simulink model "NPC_grid_tied"  (R2020a)
settings: Solver=ode8  StartTime=0.0  StopTime=0.1  FixedStep=1e-6  RelTol=1e-3
libraries: powerlib x31, simulink x6
(part 1 of 2)
settings Model: Creator=Administrator  LastModifiedBy=captaincc
settings DataIOCC: ReturnWorkspaceOutputs=off
settings DebuggingCC: ArithmeticOperatorsInVariantConditions=warning
settings SFSimCC: CustomCodeUndefinedFunction=UseInterfaceOnly

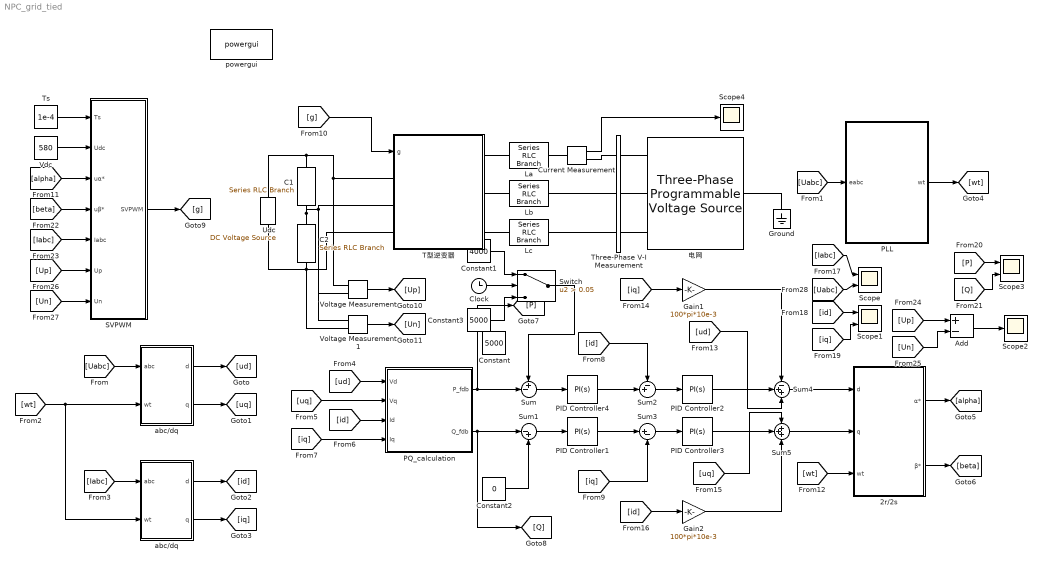
== system NPC_grid_tied ==
  2r/2s : Subsystem
  Add : Sum  Inputs=+-
  C1 : powerlib/Elements/Series RLC Branch  LConnTagsString=__new0  RConnTagsString=__new0  BranchType=RC  Resistance=1e-3  Inductance=1e-3  SetiL0=off  InitialCurrent=0  Capacitance=600e-6  Setx0=off  InitialVoltage=0  Measurements=None
  C2 : powerlib/Elements/Series RLC Branch  LConnTagsString=__new0  RConnTagsString=__new0  BranchType=RC  Resistance=1e-3  Inductance=1e-3  SetiL0=off  InitialCurrent=0  Capacitance=600e-6  Setx0=off  InitialVoltage=0  Measurements=None
  Clock : Clock
  Constant : Constant  Value=5000
  Constant1 : Constant  Value=4000
  Constant2 : Constant  Value=0
  Constant3 : Constant  Value=5000
  Current Measurement : powerlib/Measurements/Current Measurement  PhasorSimulation=off  OutputType=Complex  PSBequivalent=0
  Gain1 : Gain  Gain=100*pi*10e-3
  Gain2 : Gain  Gain=100*pi*10e-3
  Ground : powerlib/Elements/Ground  LConnTagsString=a
  La : powerlib/Elements/Series RLC Branch  LConnTagsString=__new0  RConnTagsString=__new0  BranchType=L  Resistance=1  Inductance=10e-3  SetiL0=off  InitialCurrent=0  Capacitance=1e-6  Setx0=off  InitialVoltage=0  Measurements=None
  Lb : powerlib/Elements/Series RLC Branch  LConnTagsString=__new0  RConnTagsString=__new0  BranchType=L  Resistance=1  Inductance=10e-3  SetiL0=off  InitialCurrent=0  Capacitance=1e-6  Setx0=off  InitialVoltage=0  Measurements=None
  Lc : powerlib/Elements/Series RLC Branch  LConnTagsString=__new0  RConnTagsString=__new0  BranchType=L  Resistance=1  Inductance=10e-3  SetiL0=off  InitialCurrent=0  Capacitance=1e-6  Setx0=off  InitialVoltage=0  Measurements=None
  PID Controller1 : simulink/Continuous/PID Controller  Controller=PI  Form=Parallel  TimeDomain=Continuous-time  UseExternalTs=off  SampleTime=-1  IntegratorMethod=Forward Euler  FilterMethod=Forward Euler  ControllerParametersSource=internal  P=0.0014  I=1.0395  D=0  UseFilter=on  N=100  TunerSelectOption=Transfer Function Based (PID Tuner App)  InitialConditionSource=internal  InitialConditionForIntegrator=0  InitialConditionForFilter=0  DifferentiatorICPrevScaledInput=0  ExternalReset=none  TrackingMode=off  Kt=1  LimitOutput=off  UpperSaturationLimit=inf  LowerSaturationLimit=-inf  LinearizeAsGain=on  AntiWindupMode=none  Kb=1  POutMin=[]  POutMax=[]  IOutMin=[]  IOutMax=[]  DOutMin=[]  DOutMax=[]  NOutMin=[]  NOutMax=[]  SumOutMin=[]  SumOutMax=[]  SaturationOutMin=[]  SaturationOutMax=[]  PParamMin=[]  PParamMax=[]  IParamMin=[]  IParamMax=[]  DParamMin=[]  DParamMax=[]  NParamMin=[]  NParamMax=[]  KbParamMin=[]  KbParamMax=[]  KtParamMin=[]  KtParamMax=[]  KbOutMin=[]  KbOutMax=[]  KtOutMin=[]  KtOutMax=[]  IntegratorOutMin=[]  IntegratorOutMax=[]  FilterOutMin=[]  FilterOutMax=[]  SumI1OutMin=[]  SumI1OutMax=[]  SumI2OutMin=[]  SumI2OutMax=[]  SumI3OutMin=[]  SumI3OutMax=[]  SumI4OutMin=[]  SumI4OutMax=[]  SumDOutMin=[]  SumDOutMax=[]  DifferentiatorOutMin=[]  DifferentiatorOutMax=[]  FilterDiffOutCoefMin=[]  FilterDiffOutCoefMax=[]  ReciprocalOutMin=[]  ReciprocalOutMax=[]  SumDenOutMin=[]  SumDenOutMax=[]  SumNumOutMin=[]  SumNumOutMax=[]  DivideOutMin=[]  DivideOutMax=[]  UdiffTsProdOutMin=[]  UdiffTsProdOutMax=[]  NTsProdOutMin=[]  NTsProdOutMax=[]  UintegralTsProdOutMin=[]  UintegralTsProdOutMax=[]  UngainTsProdOutMin=[]  UngainTsProdOutMax=[]  IntegratorContinuousStateAttributes=''  IntegratorStateMustResolveToSignalObject=off  IntegratorRTWStateStorageClass=Auto  FilterContinuousStateAttributes=''  FilterStateMustResolveToSignalObject=off  FilterRTWStateStorageClass=Auto  ParallelPVariant=InternalParameters  IdealPVariant=Disabled  IVariant=InternalParameters  DVariant=Disabled  IntegratorVariant=Continuous  SatVariant=Disabled  AWVariant=Passthrough  PCopyVariant=Disabled  TRVariant=Disabled  FdbkBlocksVariant=Forward  IdealPFdbkVariant=Disabled  SatFdbkVariant=Disabled  DerivativeFilterVariant=Disabled  NVariant=Disabled  NCopyVariant=Disabled_SignalSpec  FilterICVariant=Disabled  IntegratorICVariant=InternalICs  ExternalResetVariant=Disabled  TRSumVariant=Passthrough  SumFdbkVariant=Disabled  SumVariant=Sum_PI  TsampFilterVariant=InternalTs  TsampNgainVariant=Passthrough  TsampIntegralVariant=Passthrough
  PID Controller2 : simulink/Continuous/PID Controller  Controller=PI  Form=Parallel  TimeDomain=Continuous-time  UseExternalTs=off  SampleTime=-1  IntegratorMethod=Forward Euler  FilterMethod=Forward Euler  ControllerParametersSource=internal  P=33  I=333  D=0  UseFilter=on  N=100  TunerSelectOption=Transfer Function Based (PID Tuner App)  InitialConditionSource=internal  InitialConditionForIntegrator=0  InitialConditionForFilter=0  DifferentiatorICPrevScaledInput=0  ExternalReset=none  TrackingMode=off  Kt=1  LimitOutput=off  UpperSaturationLimit=inf  LowerSaturationLimit=-inf  LinearizeAsGain=on  AntiWindupMode=none  Kb=1  POutMin=[]  POutMax=[]  IOutMin=[]  IOutMax=[]  DOutMin=[]  DOutMax=[]  NOutMin=[]  NOutMax=[]  SumOutMin=[]  SumOutMax=[]  SaturationOutMin=[]  SaturationOutMax=[]  PParamMin=[]  PParamMax=[]  IParamMin=[]  IParamMax=[]  DParamMin=[]  DParamMax=[]  NParamMin=[]  NParamMax=[]  KbParamMin=[]  KbParamMax=[]  KtParamMin=[]  KtParamMax=[]  KbOutMin=[]  KbOutMax=[]  KtOutMin=[]  KtOutMax=[]  IntegratorOutMin=[]  IntegratorOutMax=[]  FilterOutMin=[]  FilterOutMax=[]  SumI1OutMin=[]  SumI1OutMax=[]  SumI2OutMin=[]  SumI2OutMax=[]  SumI3OutMin=[]  SumI3OutMax=[]  SumI4OutMin=[]  SumI4OutMax=[]  SumDOutMin=[]  SumDOutMax=[]  DifferentiatorOutMin=[]  DifferentiatorOutMax=[]  FilterDiffOutCoefMin=[]  FilterDiffOutCoefMax=[]  ReciprocalOutMin=[]  ReciprocalOutMax=[]  SumDenOutMin=[]  SumDenOutMax=[]  SumNumOutMin=[]  SumNumOutMax=[]  DivideOutMin=[]  DivideOutMax=[]  UdiffTsProdOutMin=[]  UdiffTsProdOutMax=[]  NTsProdOutMin=[]  NTsProdOutMax=[]  UintegralTsProdOutMin=[]  UintegralTsProdOutMax=[]  UngainTsProdOutMin=[]  UngainTsProdOutMax=[]  IntegratorContinuousStateAttributes=''  IntegratorStateMustResolveToSignalObject=off  IntegratorRTWStateStorageClass=Auto  FilterContinuousStateAttributes=''  FilterStateMustResolveToSignalObject=off  FilterRTWStateStorageClass=Auto  ParallelPVariant=InternalParameters  IdealPVariant=Disabled  IVariant=InternalParameters  DVariant=Disabled  IntegratorVariant=Continuous  SatVariant=Disabled  AWVariant=Passthrough  PCopyVariant=Disabled  TRVariant=Disabled  FdbkBlocksVariant=Forward  IdealPFdbkVariant=Disabled  SatFdbkVariant=Disabled  DerivativeFilterVariant=Disabled  NVariant=Disabled  NCopyVariant=Disabled_SignalSpec  FilterICVariant=Disabled  IntegratorICVariant=InternalICs  ExternalResetVariant=Disabled  TRSumVariant=Passthrough  SumFdbkVariant=Disabled  SumVariant=Sum_PI  TsampFilterVariant=InternalTs  TsampNgainVariant=Passthrough  TsampIntegralVariant=Passthrough
  PID Controller3 : simulink/Continuous/PID Controller  Controller=PI  Form=Parallel  TimeDomain=Continuous-time  UseExternalTs=off  SampleTime=-1  IntegratorMethod=Forward Euler  FilterMethod=Forward Euler  ControllerParametersSource=internal  P=33  I=333  D=0  UseFilter=on  N=100  TunerSelectOption=Transfer Function Based (PID Tuner App)  InitialConditionSource=internal  InitialConditionForIntegrator=0  InitialConditionForFilter=0  DifferentiatorICPrevScaledInput=0  ExternalReset=none  TrackingMode=off  Kt=1  LimitOutput=off  UpperSaturationLimit=inf  LowerSaturationLimit=-inf  LinearizeAsGain=on  AntiWindupMode=none  Kb=1  POutMin=[]  POutMax=[]  IOutMin=[]  IOutMax=[]  DOutMin=[]  DOutMax=[]  NOutMin=[]  NOutMax=[]  SumOutMin=[]  SumOutMax=[]  SaturationOutMin=[]  SaturationOutMax=[]  PParamMin=[]  PParamMax=[]  IParamMin=[]  IParamMax=[]  DParamMin=[]  DParamMax=[]  NParamMin=[]  NParamMax=[]  KbParamMin=[]  KbParamMax=[]  KtParamMin=[]  KtParamMax=[]  KbOutMin=[]  KbOutMax=[]  KtOutMin=[]  KtOutMax=[]  IntegratorOutMin=[]  IntegratorOutMax=[]  FilterOutMin=[]  FilterOutMax=[]  SumI1OutMin=[]  SumI1OutMax=[]  SumI2OutMin=[]  SumI2OutMax=[]  SumI3OutMin=[]  SumI3OutMax=[]  SumI4OutMin=[]  SumI4OutMax=[]  SumDOutMin=[]  SumDOutMax=[]  DifferentiatorOutMin=[]  DifferentiatorOutMax=[]  FilterDiffOutCoefMin=[]  FilterDiffOutCoefMax=[]  ReciprocalOutMin=[]  ReciprocalOutMax=[]  SumDenOutMin=[]  SumDenOutMax=[]  SumNumOutMin=[]  SumNumOutMax=[]  DivideOutMin=[]  DivideOutMax=[]  UdiffTsProdOutMin=[]  UdiffTsProdOutMax=[]  NTsProdOutMin=[]  NTsProdOutMax=[]  UintegralTsProdOutMin=[]  UintegralTsProdOutMax=[]  UngainTsProdOutMin=[]  UngainTsProdOutMax=[]  IntegratorContinuousStateAttributes=''  IntegratorStateMustResolveToSignalObject=off  IntegratorRTWStateStorageClass=Auto  FilterContinuousStateAttributes=''  FilterStateMustResolveToSignalObject=off  FilterRTWStateStorageClass=Auto  ParallelPVariant=InternalParameters  IdealPVariant=Disabled  IVariant=InternalParameters  DVariant=Disabled  IntegratorVariant=Continuous  SatVariant=Disabled  AWVariant=Passthrough  PCopyVariant=Disabled  TRVariant=Disabled  FdbkBlocksVariant=Forward  IdealPFdbkVariant=Disabled  SatFdbkVariant=Disabled  DerivativeFilterVariant=Disabled  NVariant=Disabled  NCopyVariant=Disabled_SignalSpec  FilterICVariant=Disabled  IntegratorICVariant=InternalICs  ExternalResetVariant=Disabled  TRSumVariant=Passthrough  SumFdbkVariant=Disabled  SumVariant=Sum_PI  TsampFilterVariant=InternalTs  TsampNgainVariant=Passthrough  TsampIntegralVariant=Passthrough
  PID Controller4 : simulink/Continuous/PID Controller  Controller=PI  Form=Parallel  TimeDomain=Continuous-time  UseExternalTs=off  SampleTime=-1  IntegratorMethod=Forward Euler  FilterMethod=Forward Euler  ControllerParametersSource=internal  P=0.0014  I=1.0395  D=0  UseFilter=on  N=100  TunerSelectOption=Transfer Function Based (PID Tuner App)  InitialConditionSource=internal  InitialConditionForIntegrator=0  InitialConditionForFilter=0  DifferentiatorICPrevScaledInput=0  ExternalReset=none  TrackingMode=off  Kt=1  LimitOutput=off  UpperSaturationLimit=inf  LowerSaturationLimit=-inf  LinearizeAsGain=on  AntiWindupMode=none  Kb=1  POutMin=[]  POutMax=[]  IOutMin=[]  IOutMax=[]  DOutMin=[]  DOutMax=[]  NOutMin=[]  NOutMax=[]  SumOutMin=[]  SumOutMax=[]  SaturationOutMin=[]  SaturationOutMax=[]  PParamMin=[]  PParamMax=[]  IParamMin=[]  IParamMax=[]  DParamMin=[]  DParamMax=[]  NParamMin=[]  NParamMax=[]  KbParamMin=[]  KbParamMax=[]  KtParamMin=[]  KtParamMax=[]  KbOutMin=[]  KbOutMax=[]  KtOutMin=[]  KtOutMax=[]  IntegratorOutMin=[]  IntegratorOutMax=[]  FilterOutMin=[]  FilterOutMax=[]  SumI1OutMin=[]  SumI1OutMax=[]  SumI2OutMin=[]  SumI2OutMax=[]  SumI3OutMin=[]  SumI3OutMax=[]  SumI4OutMin=[]  SumI4OutMax=[]  SumDOutMin=[]  SumDOutMax=[]  DifferentiatorOutMin=[]  DifferentiatorOutMax=[]  FilterDiffOutCoefMin=[]  FilterDiffOutCoefMax=[]  ReciprocalOutMin=[]  ReciprocalOutMax=[]  SumDenOutMin=[]  SumDenOutMax=[]  SumNumOutMin=[]  SumNumOutMax=[]  DivideOutMin=[]  DivideOutMax=[]  UdiffTsProdOutMin=[]  UdiffTsProdOutMax=[]  NTsProdOutMin=[]  NTsProdOutMax=[]  UintegralTsProdOutMin=[]  UintegralTsProdOutMax=[]  UngainTsProdOutMin=[]  UngainTsProdOutMax=[]  IntegratorContinuousStateAttributes=''  IntegratorStateMustResolveToSignalObject=off  IntegratorRTWStateStorageClass=Auto  FilterContinuousStateAttributes=''  FilterStateMustResolveToSignalObject=off  FilterRTWStateStorageClass=Auto  ParallelPVariant=InternalParameters  IdealPVariant=Disabled  IVariant=InternalParameters  DVariant=Disabled  IntegratorVariant=Continuous  SatVariant=Disabled  AWVariant=Passthrough  PCopyVariant=Disabled  TRVariant=Disabled  FdbkBlocksVariant=Forward  IdealPFdbkVariant=Disabled  SatFdbkVariant=Disabled  DerivativeFilterVariant=Disabled  NVariant=Disabled  NCopyVariant=Disabled_SignalSpec  FilterICVariant=Disabled  IntegratorICVariant=InternalICs  ExternalResetVariant=Disabled  TRSumVariant=Passthrough  SumFdbkVariant=Disabled  SumVariant=Sum_PI  TsampFilterVariant=InternalTs  TsampNgainVariant=Passthrough  TsampIntegralVariant=Passthrough
  PLL : Subsystem
  PQ_calculation : Subsystem
  SVPWM : Subsystem
  Scope : Scope  NumInputPorts=2
  Scope1 : Scope  NumInputPorts=2
  Scope2 : Scope
  Scope3 : Scope  NumInputPorts=2
  Scope4 : Scope
  Sum : Sum  Inputs=+-|
  Sum1 : Sum  Inputs=|-+
  Sum2 : Sum  Inputs=-+|
  Sum3 : Sum  Inputs=|+-
  Sum4 : Sum  Inputs=-++
  Sum5 : Sum  Inputs=+++
  Switch : Switch  Criteria=u2 > Threshold  Threshold=0.05
  Three-Phase V-I Measurement : powerlib/Measurements/Three-Phase V-I Measurement  VoltageMeasurement=phase-to-ground  SetLabelV=on  LabelV=Uabc  Vpu=off  VpuLL=off  CurrentMeasurement=yes  SetLabelI=on  LabelI=Iabc  Ipu=off  Pbase=100e6  Vbase=500e3  OutputType=Complex  PhasorSimulation=off  PSBequivalent=0
  Ts : Constant  Value=1e-4
  T型逆变器 : Subsystem
  Udc : powerlib/Electrical Sources/DC Voltage Source  Amplitude=580  Measurements=None
  Vdc : Constant  Value=580
  Voltage Measurement : powerlib/Measurements/Voltage Measurement  PhasorSimulation=off  OutputType=Complex  PSBequivalent=0
  Voltage Measurement1 : powerlib/Measurements/Voltage Measurement  PhasorSimulation=off  OutputType=Complex  PSBequivalent=0
  abc/dq : Subsystem
  "abc/dq " : Subsystem
  powergui : powerlib/powergui  Priority=1  SimulationMode=Continuous  SampleTime=1e-6  frequency=60  Iterations=50  frequencyindice=0  Pbase=100e6  ErrMax=1e-4  UnitsV=kV  UnitsW=MW  buscounter=0  FunctionMessages=off  echomessages=off  EnableUseOfTLC=off  CurrentSourceSwitches=off  DisableSnubberDevices=off  DisableRonSwitches=off  DisableVfSwitches=off  DisplayEquations=off  AutomaticDiscreteSolvers=off  SolverType=Tustin/Backward Euler (TBE)  Interpol=off  ExternalGateDelay=off  methode=off  Ts=100  x0status=blocks  SPID=off  SwTol=0  HookPort=off  NonlinearTolerance=1e-4  nMaxIteration=100  ContinueOnMaxIteration=off  RestoreLinks=warning  ResistiveCurrentMeasurement=off  Frange=[0:2:500]  Ylog=off  Xlog=on  ShowGrid=off  save=off  variable=ZData  structure=Ia  ZoomFFT=off  StartTime=0.03  cycles=2  DisplayStyle=1  fundamental=50  FreqAxis=off  MaxFrequency=1000  frequencyindicesteady=1  RmsSteady=1  display=off
  电网 : powerlib/Electrical Sources/Three-Phase Programmable Voltage Source  PositiveSequence=[220*sqrt(3) 0 50]  VariationEntity=None  VariationType=Step  VariationTypeAlt=Step  VariationStep=0.5  VariationRate=10  VariationMagnitude=0.3  VariationFrequency=2  VariationTiming=[1 2]  VariationPhaseA=off  Amplitudes=[1 0.8 1.2 1.0]  TimeValues=[0 0.1 0.15 0.2]  HarmonicGeneration=off  HarmonicA=[3 0.2 -25 0]  HarmonicB=[2 0.15 35 2]  Timing="[0.05  3]"  BusType=swing  Pref=10000  Qref=0  Qmin=-inf  Qmax=inf
  wires:
  [Uabc] -> PLL/1(eabc)
  PLL/1(wt) -> [wt]
  [ud] -> PQ_calculation/1(Vd)
  [uq] -> PQ_calculation/2(Vq)
  [id] -> PQ_calculation/3(Id)
  [iq] -> PQ_calculation/4(Iq)
  PQ_calculation/2(Q_fdb) -> Sum1/1, [Q]
  PQ_calculation/1(P_fdb) -> Sum/2, [P]
  Constant2/1 -> Sum1/2
  PID Controller4/1 -> Sum2/2
  PID Controller1/1 -> Sum3/1
  [id] -> Sum2/1
  [iq] -> Sum3/2
  Sum2/1 -> PID Controller2/1
  Sum3/1 -> PID Controller3/1
  [wt] -> 2r/2s/3(wt)
  2r/2s/1(α*) -> [alpha]
  2r/2s/2(β*) -> [beta]
  [wt] -> "abc/dq "/2(wt), abc/dq/2(wt)
  [Iabc] -> "abc/dq "/1(abc)
  abc/dq/2(q) -> [uq]
  abc/dq/1(d) -> [ud]
  [Uabc] -> abc/dq/1(abc)
  "abc/dq "/2(q) -> [iq]
  "abc/dq "/1(d) -> [id]
  [ud] -> Sum4/3
  PID Controller2/1 -> Sum4/2
  [iq] -> Gain1/1
  Gain1/1 -> Sum4/1
  PID Controller3/1 -> Sum5/2
  Gain2/1 -> Sum5/3
  [uq] -> Sum5/1
  [id] -> Gain2/1
  Current Measurement/1 -> Scope4/1
  [id] -> Scope1/1
  [iq] -> Scope1/2
  [P] -> Scope3/1
  [Q] -> Scope3/2
  Sum4/1 -> 2r/2s/1(d)
  Sum5/1 -> 2r/2s/2(q)
  Sum/1 -> PID Controller4/1
  Sum1/1 -> PID Controller1/1
  Ts/1 -> SVPWM/1(Ts)
  Vdc/1 -> SVPWM/2(Udc)
  [g] -> T型逆变器/1(g)
  SVPWM/1(SVPWM) -> [g]
  [alpha] -> SVPWM/3(uα*)
  [beta] -> SVPWM/4(uβ*)
  [Iabc] -> Scope/1
  [Iabc] -> SVPWM/5(Iabc)
  Voltage Measurement/1 -> [Up]
  Voltage Measurement1/1 -> [Un]
  [Up] -> Add/1
  [Un] -> Add/2
  Add/1 -> Scope2/1
  [Up] -> SVPWM/6(Up)
  [Un] -> SVPWM/7(Un)
  [Uabc] -> Scope/2
  Switch/1 -> Sum/1
  Clock/1 -> Switch/2
  Constant3/1 -> Switch/3
  Constant1/1 -> Switch/1
  connections:
  T型逆变器/RConn1 -- La/LConn1
  电网/RConn1 -- Three-Phase V-I Measurement/RConn1
  Three-Phase V-I Measurement/LConn2 -- Lb/RConn1
  Three-Phase V-I Measurement/LConn3 -- Lc/RConn1
  T型逆变器/RConn2 -- Lb/LConn1
  T型逆变器/RConn3 -- Lc/LConn1
  电网/RConn2 -- Three-Phase V-I Measurement/RConn2
  电网/RConn3 -- Three-Phase V-I Measurement/RConn3
  Ground/LConn1 -- 电网/LConn1
  Current Measurement/LConn1 -- La/RConn1
  Current Measurement/RConn1 -- Three-Phase V-I Measurement/LConn1
  Udc/LConn1 -- Voltage Measurement1/LConn2 -- C2/RConn1 -- T型逆变器/LConn3
  C2/LConn1 -- Voltage Measurement1/LConn1 -- Voltage Measurement/LConn2 -- T型逆变器/LConn2 -- C1/RConn1
  C1/LConn1 -- Udc/RConn1 -- Voltage Measurement/LConn1 -- T型逆变器/LConn1

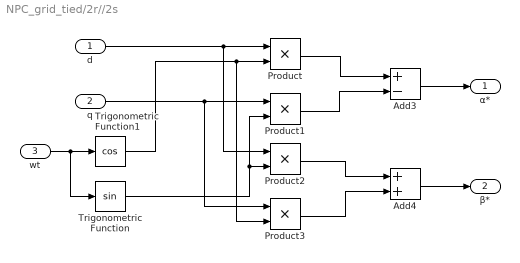
== system NPC_grid_tied/2r//2s ==
  d : Inport
  q : Inport  Port=2
  wt : Inport  Port=3
  Add3 : Sum  Inputs=+-
  Add4 : Sum
  Product{,1..3} (4 alike) : Product
  Trigonometric Function : Trigonometry
  Trigonometric Function1 : Trigonometry  Operator=cos
  α* : Outport  VectorParamsAs1DForOutWhenUnconnected=off
  β* : Outport  Port=2  VectorParamsAs1DForOutWhenUnconnected=off
  wires:
  q/1 -> Product3/1, Product1/1
  Trigonometric Function/1 -> Product1/2, Product2/2
  Trigonometric Function1/1 -> Product3/2, Product/2
  d/1 -> Product2/1, Product/1
  Product2/1 -> Add4/1
  Product/1 -> Add3/1
  Product1/1 -> Add3/2
  Product3/1 -> Add4/2
  Add3/1 -> α*/1
  Add4/1 -> β*/1
  wt/1 -> Trigonometric Function/1, Trigonometric Function1/1

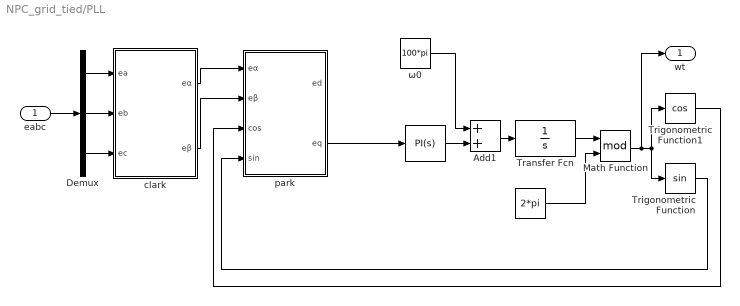
== system NPC_grid_tied/PLL ==
  eabc : Inport
  " " : Constant  Value=2*pi
  " " : simulink/Continuous/PID Controller  Controller=PI  Form=Parallel  TimeDomain=Continuous-time  UseExternalTs=off  SampleTime=-1  IntegratorMethod=Trapezoidal  FilterMethod=Forward Euler  ControllerParametersSource=internal  P=0.826  I=82.7  D=0  UseFilter=on  N=100  TunerSelectOption=Transfer Function Based (PID Tuner App)  InitialConditionSource=internal  InitialConditionForIntegrator=0  InitialConditionForFilter=0  DifferentiatorICPrevScaledInput=0  ExternalReset=none  TrackingMode=off  Kt=1  LimitOutput=off  UpperSaturationLimit=inf  LowerSaturationLimit=-inf  LinearizeAsGain=off  AntiWindupMode=none  Kb=1  POutMin=[]  POutMax=[]  IOutMin=[]  IOutMax=[]  DOutMin=[]  DOutMax=[]  NOutMin=[]  NOutMax=[]  SumOutMin=[]  SumOutMax=[]  SaturationOutMin=[]  SaturationOutMax=[]  PParamMin=[]  PParamMax=[]  IParamMin=[]  IParamMax=[]  DParamMin=[]  DParamMax=[]  NParamMin=[]  NParamMax=[]  KbParamMin=[]  KbParamMax=[]  KtParamMin=[]  KtParamMax=[]  KbOutMin=[]  KbOutMax=[]  KtOutMin=[]  KtOutMax=[]  IntegratorOutMin=[]  IntegratorOutMax=[]  FilterOutMin=[]  FilterOutMax=[]  SumI1OutMin=[]  SumI1OutMax=[]  SumI2OutMin=[]  SumI2OutMax=[]  SumI3OutMin=[]  SumI3OutMax=[]  SumI4OutMin=[]  SumI4OutMax=[]  SumDOutMin=[]  SumDOutMax=[]  DifferentiatorOutMin=[]  DifferentiatorOutMax=[]  FilterDiffOutCoefMin=[]  FilterDiffOutCoefMax=[]  ReciprocalOutMin=[]  ReciprocalOutMax=[]  SumDenOutMin=[]  SumDenOutMax=[]  SumNumOutMin=[]  SumNumOutMax=[]  DivideOutMin=[]  DivideOutMax=[]  UdiffTsProdOutMin=[]  UdiffTsProdOutMax=[]  NTsProdOutMin=[]  NTsProdOutMax=[]  UintegralTsProdOutMin=[]  UintegralTsProdOutMax=[]  UngainTsProdOutMin=[]  UngainTsProdOutMax=[]  IntegratorContinuousStateAttributes=''  IntegratorStateMustResolveToSignalObject=off  IntegratorRTWStateStorageClass=Auto  FilterContinuousStateAttributes=''  FilterStateMustResolveToSignalObject=off  FilterRTWStateStorageClass=Auto  ParallelPVariant=InternalParameters  IdealPVariant=Disabled  IVariant=InternalParameters  DVariant=Disabled  IntegratorVariant=Continuous  SatVariant=Disabled  AWVariant=Passthrough  PCopyVariant=Disabled  TRVariant=Disabled  FdbkBlocksVariant=Forward  IdealPFdbkVariant=Disabled  SatFdbkVariant=Disabled  DerivativeFilterVariant=Disabled  NVariant=Disabled  NCopyVariant=Disabled_SignalSpec  FilterICVariant=Disabled  IntegratorICVariant=InternalICs  ExternalResetVariant=Disabled  TRSumVariant=Passthrough  SumFdbkVariant=Disabled  SumVariant=Sum_PI  TsampFilterVariant=InternalTs  TsampNgainVariant=Passthrough  TsampIntegralVariant=Passthrough
  Add1 : Sum
  Demux : Demux  Outputs=3
  Math Function : Math  Operator=mod  SignedPower=on  SaturateOnIntegerOverflow=on
  Transfer Fcn : TransferFcn  Denominator=[1 0]
  Trigonometric Function : Trigonometry
  Trigonometric Function1 : Trigonometry  Operator=cos
  clark : Subsystem
  park : Subsystem
  ω0 : Constant  Value=100*pi
  wt : Outport  VectorParamsAs1DForOutWhenUnconnected=off
  wires:
  Demux/2 -> clark/2(eb)
  Demux/1 -> clark/1(ea)
  Trigonometric Function/1 -> park/4(sin)
  clark/1(eα) -> park/1(eα)
  Trigonometric Function1/1 -> park/3(cos)
  Transfer Fcn/1 -> Math Function/1
  " "/1 -> Add1/2
  ω0/1 -> Add1/1
  Add1/1 -> Transfer Fcn/1
  clark/2(eβ) -> park/2(eβ)
  Demux/3 -> clark/3(ec)
  eabc/1 -> Demux/1
  park/2(eq) -> " "/1
  " "/1 -> Math Function/2
  Math Function/1 -> wt/1, Trigonometric Function/1, Trigonometric Function1/1

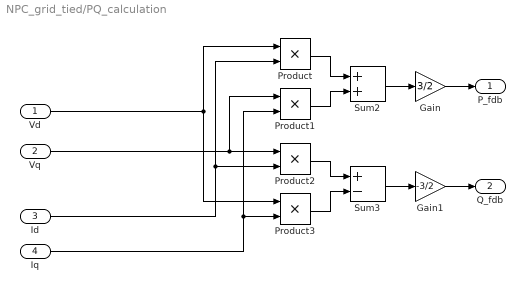
== system NPC_grid_tied/PQ_calculation ==
  Vd : Inport
  Vq : Inport  Port=2
  Id : Inport  Port=3
  Iq : Inport  Port=4
  Gain : Gain  Gain=3/2
  Gain1 : Gain  Gain=-3/2
  Product{,1..3} (4 alike) : Product
  Sum2 : Sum
  Sum3 : Sum  Inputs=+-
  P_fdb : Outport  VectorParamsAs1DForOutWhenUnconnected=off
  Q_fdb : Outport  Port=2  VectorParamsAs1DForOutWhenUnconnected=off
  wires:
  Product2/1 -> Sum3/1
  Iq/1 -> Product3/2, Product1/2
  Product3/1 -> Sum3/2
  Vq/1 -> Product1/1, Product2/1
  Id/1 -> Product2/2, Product/2
  Product/1 -> Sum2/1
  Vd/1 -> Product3/1, Product/1
  Product1/1 -> Sum2/2
  Gain/1 -> P_fdb/1
  Sum2/1 -> Gain/1
  Gain1/1 -> Q_fdb/1
  Sum3/1 -> Gain1/1

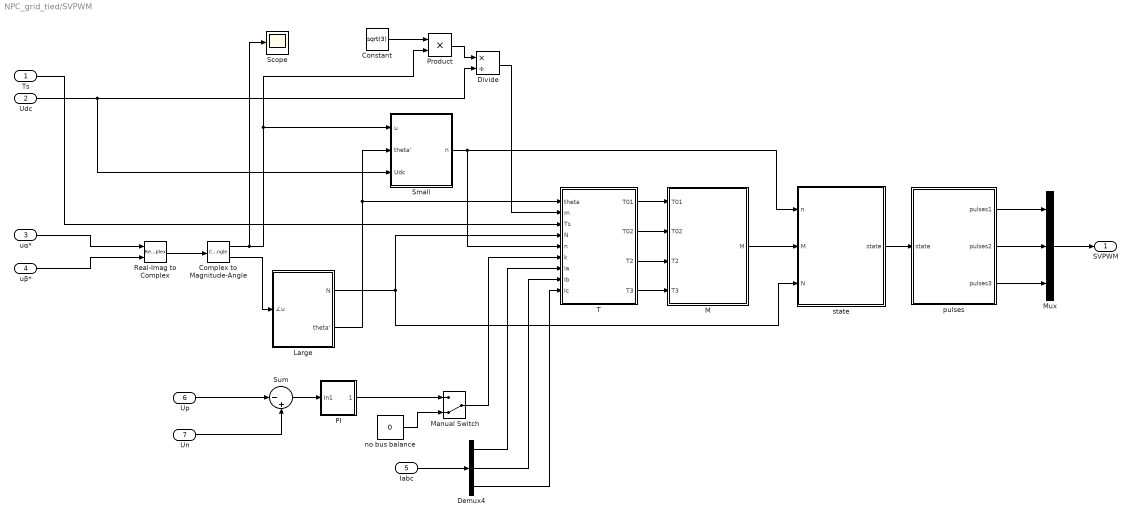
== system NPC_grid_tied/SVPWM ==
  Ts : Inport
  Udc : Inport  Port=2
  uα* : Inport  Port=3
  uβ* : Inport  Port=4
  Iabc : Inport  Port=5
  Up : Inport  Port=6
  Un : Inport  Port=7
  Complex to Magnitude-Angle : ComplexToMagnitudeAngle
  Constant : Constant  Value=sqrt(3)
  Demux4 : Demux  Outputs=3
  Divide : Product  Inputs=*/
  Large : Subsystem
  M : Subsystem
  Manual Switch : ManualSwitch  CurrentSetting=0
  Mux : Mux  Inputs=3
  PI : Subsystem
  Product : Product
  Real-Imag to Complex : RealImagToComplex
  Scope : Scope
  Small : Subsystem
  Sum : Sum  Inputs=|-+
  T : MATLAB Function  TreatAsAtomicUnit=on
  no bus balance : Constant  Value=0
  pulses : Subsystem
  state : Subsystem
  SVPWM : Outport  VectorParamsAs1DForOutWhenUnconnected=off
  wires:
  Udc/1 -> Divide/2, Small/3(Udc)
  Large/2(theta') -> T/1(theta), Small/2(theta')
  Product/1 -> Divide/1
  Complex to Magnitude-Angle/2 -> Large/1(∠u)
  Complex to Magnitude-Angle/1 -> Scope/1, Product/2, Small/1(u)
  Constant/1 -> Product/1
  pulses/1(pulses1) -> Mux/1
  pulses/2(pulses2) -> Mux/2
  pulses/3(pulses3) -> Mux/3
  state/1(state) -> pulses/1(state)
  Mux/1 -> SVPWM/1
  Real-Imag to Complex/1 -> Complex to Magnitude-Angle/1
  uα*/1 -> Real-Imag to Complex/1
  uβ*/1 -> Real-Imag to Complex/2
  Ts/1 -> T/3(Ts)
  PI/1(Out1) -> Manual Switch/1
  Demux4/1 -> T/7(Ia)
  Manual Switch/1 -> T/6(k)
  Large/1(N) -> T/4(N), state/3(N)
  T/1(T01) -> M/1(T01)
  Small/1(n) -> T/5(n), state/1(n)
  Divide/1 -> T/2(m)
  Demux4/3 -> T/9(Ic)
  Iabc/1 -> Demux4/1
  T/2(T02) -> M/2(T02)
  T/3(T2) -> M/3(T2)
  no bus balance/1 -> Manual Switch/2
  Demux4/2 -> T/8(Ib)
  T/4(T3) -> M/4(T3)
  M/1(M) -> state/2(M)
  Sum/1 -> PI/1(In1)
  Up/1 -> Sum/1
  Un/1 -> Sum/2

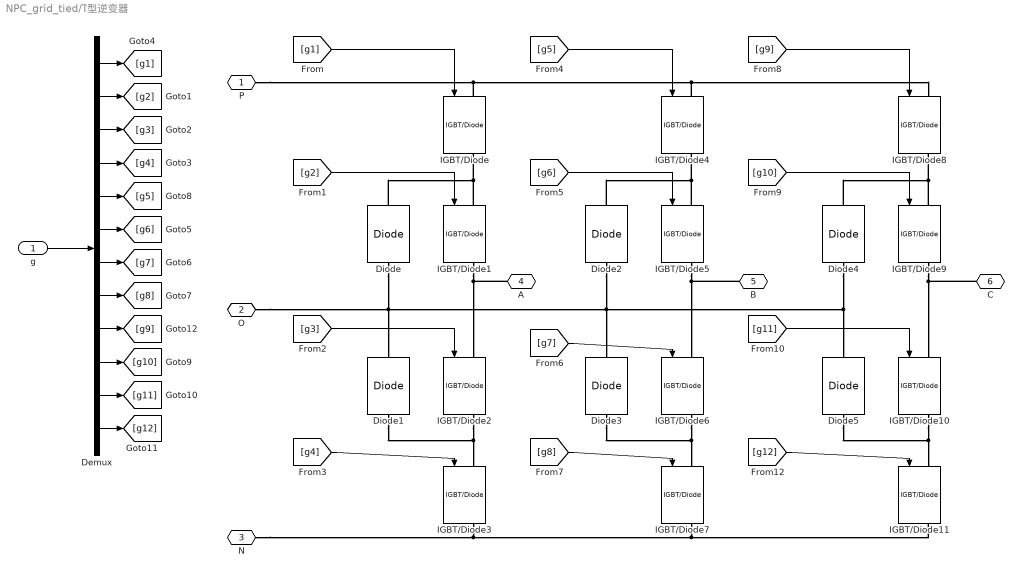
== system NPC_grid_tied/T型逆变器 ==
  g : Inport
  Demux : Demux  Outputs=12
  Diode{,1..5} (6 alike) : powerlib/Power Electronics/Diode  Ron=0.001  Lon=0  Vf=0.8  IC=0  UseSnubber=0  Rs=500  Cs=250e-9  Measurements=off
  IGBT/Diode{,1..11} (12 alike) : powerlib/Power Electronics/IGBT//Diode  Ron=1e-3  Rs=1e5  Cs=inf  Measurements=on
  P : PMIOPort  Side=Left
  O : PMIOPort  Port=2  Side=Left
  N : PMIOPort  Port=3  Side=Left
  A : PMIOPort  Port=4  Side=Right
  B : PMIOPort  Port=5  Side=Right
  C : PMIOPort  Port=6  Side=Right
  wires:
  Demux/1 -> [g1]
  Demux/2 -> [g2]
  Demux/3 -> [g3]
  Demux/4 -> [g4]
  Demux/5 -> [g5]
  Demux/6 -> [g6]
  Demux/7 -> [g7]
  Demux/8 -> [g8]
  Demux/9 -> [g9]
  Demux/10 -> [g10]
  Demux/11 -> [g11]
  Demux/12 -> [g12]
  [g1] -> IGBT/Diode/1
  [g2] -> IGBT/Diode1/1
  [g3] -> IGBT/Diode2/1
  [g4] -> IGBT/Diode3/1
  [g5] -> IGBT/Diode4/1
  [g6] -> IGBT/Diode5/1
  [g7] -> IGBT/Diode6/1
  [g8] -> IGBT/Diode7/1
  [g9] -> IGBT/Diode8/1
  [g10] -> IGBT/Diode9/1
  [g11] -> IGBT/Diode10/1
  [g12] -> IGBT/Diode11/1
  g/1 -> Demux/1
  connections:
  IGBT/Diode1/LConn1 -- Diode/RConn1 -- IGBT/Diode/RConn1
  IGBT/Diode1/RConn1 -- A/RConn1 -- IGBT/Diode2/LConn1
  IGBT/Diode2/RConn1 -- Diode1/LConn1 -- IGBT/Diode3/LConn1
  IGBT/Diode6/RConn1 -- Diode3/LConn1 -- IGBT/Diode7/LConn1
  IGBT/Diode5/LConn1 -- Diode2/RConn1 -- IGBT/Diode4/RConn1
  IGBT/Diode5/RConn1 -- IGBT/Diode6/LConn1 -- B/RConn1
  IGBT/Diode10/RConn1 -- Diode5/LConn1 -- IGBT/Diode11/LConn1
  IGBT/Diode9/LConn1 -- Diode4/RConn1 -- IGBT/Diode8/RConn1
  IGBT/Diode9/RConn1 -- C/RConn1 -- IGBT/Diode10/LConn1
  Diode/LConn1 -- Diode5/RConn1 -- Diode4/LConn1 -- Diode2/LConn1 -- Diode3/RConn1 -- O/RConn1 -- Diode1/RConn1
  IGBT/Diode/LConn1 -- P/RConn1 -- IGBT/Diode4/LConn1 -- IGBT/Diode8/LConn1
  IGBT/Diode3/RConn1 -- IGBT/Diode7/RConn1 -- IGBT/Diode11/RConn1 -- N/RConn1

== system NPC_grid_tied/abc//dq ==
  abc : Inport
  wt : Inport  Port=2
  Demux : Demux  Outputs=3
  Trigonometric Function : Trigonometry
  Trigonometric Function1 : Trigonometry  Operator=cos
  clark : Subsystem
  park : Subsystem
  d : Outport  VectorParamsAs1DForOutWhenUnconnected=off
  q : Outport  Port=2  VectorParamsAs1DForOutWhenUnconnected=off
  wires:
  Demux/1 -> clark/1(ea)
  clark/1(eα) -> park/1(eα)
  Demux/2 -> clark/2(eb)
  Trigonometric Function1/1 -> park/3(cos)
  wt/1 -> Trigonometric Function/1, Trigonometric Function1/1
  Demux/3 -> clark/3(ec)
  clark/2(eβ) -> park/2(eβ)
  park/2(eq) -> q/1
  park/1(ed) -> d/1
  abc/1 -> Demux/1
  Trigonometric Function/1 -> park/4(sin)

== system NPC_grid_tied/abc//dq  ==
  abc : Inport
  wt : Inport  Port=2
  Demux : Demux  Outputs=3
  Trigonometric Function : Trigonometry
  Trigonometric Function1 : Trigonometry  Operator=cos
  clark : Subsystem
  park : Subsystem
  d : Outport  VectorParamsAs1DForOutWhenUnconnected=off
  q : Outport  Port=2  VectorParamsAs1DForOutWhenUnconnected=off
  wires:
  Demux/1 -> clark/1(ea)
  clark/1(eα) -> park/1(eα)
  Demux/2 -> clark/2(eb)
  Trigonometric Function1/1 -> park/3(cos)
  wt/1 -> Trigonometric Function/1, Trigonometric Function1/1
  Demux/3 -> clark/3(ec)
  clark/2(eβ) -> park/2(eβ)
  park/2(eq) -> q/1
  park/1(ed) -> d/1
  abc/1 -> Demux/1
  Trigonometric Function/1 -> park/4(sin)

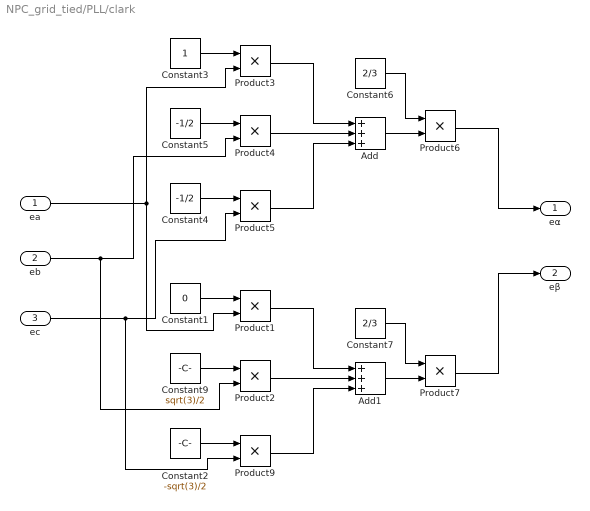
== system NPC_grid_tied/PLL/clark ==
  ea : Inport
  eb : Inport  Port=2
  ec : Inport  Port=3
  Add : Sum  Inputs=+++
  Add1 : Sum  Inputs=+++
  Constant1 : Constant  Value=0
  Constant2 : Constant  Value=-sqrt(3)/2
  Constant3 : Constant
  Constant4 : Constant  Value=-1/2
  Constant5 : Constant  Value=-1/2
  Constant6 : Constant  Value=2/3
  Constant7 : Constant  Value=2/3
  Constant9 : Constant  Value=sqrt(3)/2
  Product{1..7,9} (8 alike) : Product
  eα : Outport  VectorParamsAs1DForOutWhenUnconnected=off
  eβ : Outport  Port=2  VectorParamsAs1DForOutWhenUnconnected=off
  wires:
  Product5/1 -> Add/3
  eb/1 -> Product2/2, Product4/2
  Add1/1 -> Product7/2
  Constant7/1 -> Product7/1
  Product2/1 -> Add1/2
  Product4/1 -> Add/2
  Add/1 -> Product6/2
  Product6/1 -> eα/1
  Constant3/1 -> Product3/1
  Constant5/1 -> Product4/1
  ec/1 -> Product9/2, Product5/2
  ea/1 -> Product3/2, Product1/2
  Constant4/1 -> Product5/1
  Constant6/1 -> Product6/1
  Constant9/1 -> Product2/1
  Product3/1 -> Add/1
  Constant2/1 -> Product9/1
  Product9/1 -> Add1/3
  Product1/1 -> Add1/1
  Product7/1 -> eβ/1
  Constant1/1 -> Product1/1

== system NPC_grid_tied/PLL/park ==
  eα : Inport
  eβ : Inport  Port=2
  cos : Inport  Port=3
  sin : Inport  Port=4
  Add : Sum
  Add2 : Sum  Inputs=-+
  Product{,1..3} (4 alike) : Product
  ed : Outport  VectorParamsAs1DForOutWhenUnconnected=off
  eq : Outport  Port=2  VectorParamsAs1DForOutWhenUnconnected=off
  wires:
  Add2/1 -> eq/1
  Add/1 -> ed/1
  eα/1 -> Product2/1, Product/1
  cos/1 -> Product3/2, Product/2
  eβ/1 -> Product3/1, Product1/1
  sin/1 -> Product2/2, Product1/2
  Product/1 -> Add/1
  Product1/1 -> Add/2
  Product2/1 -> Add2/1
  Product3/1 -> Add2/2

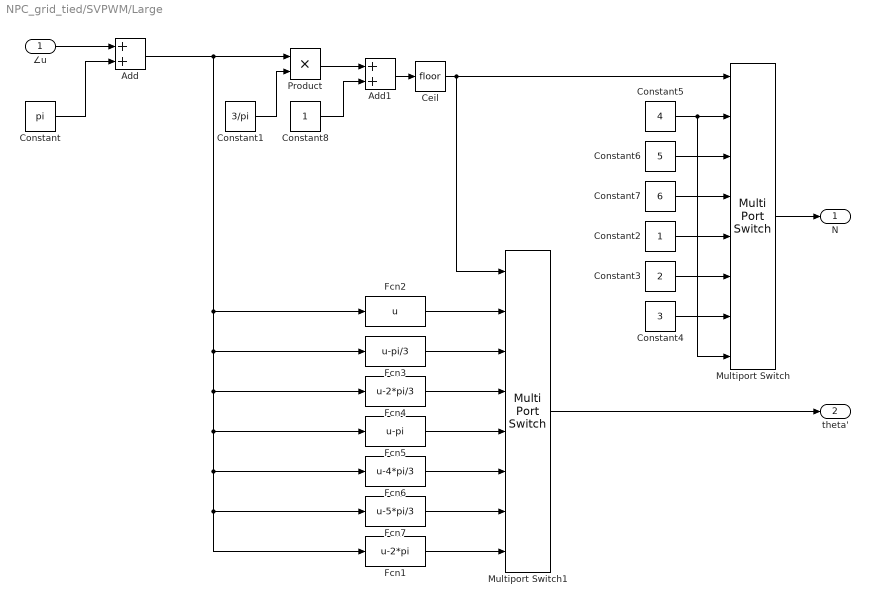
== system NPC_grid_tied/SVPWM/Large ==
  ∠u : Inport
  Add : Sum
  Add1 : Sum
  Ceil : Rounding
  Constant : Constant  Value=pi
  Constant1 : Constant  Value=3/pi
  Constant2 : Constant
  Constant3 : Constant  Value=2
  Constant4 : Constant  Value=3
  Constant5 : Constant  Value=4
  Constant6 : Constant  Value=5
  Constant7 : Constant  Value=6
  Constant8 : Constant
  Fcn1 : Fcn  Expr=u-2*pi
  Fcn2 : Fcn  Expr=u
  Fcn3 : Fcn  Expr=u-pi/3
  Fcn4 : Fcn  Expr=u-2*pi/3
  Fcn5 : Fcn  Expr=u-pi
  Fcn6 : Fcn  Expr=u-4*pi/3
  Fcn7 : Fcn  Expr=u-5*pi/3
  Multiport Switch : MultiPortSwitch  Inputs=7
  Multiport Switch1 : MultiPortSwitch  Inputs=7
  Product : Product
  N : Outport  VectorParamsAs1DForOutWhenUnconnected=off
  theta' : Outport  Port=2  VectorParamsAs1DForOutWhenUnconnected=off
  wires:
  Constant3/1 -> Multiport Switch/6
  Multiport Switch/1 -> N/1
  Constant2/1 -> Multiport Switch/5
  Constant5/1 -> Multiport Switch/8, Multiport Switch/2
  Constant7/1 -> Multiport Switch/4
  Constant4/1 -> Multiport Switch/7
  Ceil/1 -> Multiport Switch1/1, Multiport Switch/1
  Constant/1 -> Add/2
  Fcn3/1 -> Multiport Switch1/3
  Fcn4/1 -> Multiport Switch1/4
  Fcn7/1 -> Multiport Switch1/7
  Constant1/1 -> Product/2
  Constant6/1 -> Multiport Switch/3
  Fcn6/1 -> Multiport Switch1/6
  Fcn2/1 -> Multiport Switch1/2
  Fcn5/1 -> Multiport Switch1/5
  Add/1 -> Fcn2/1, Fcn3/1, Fcn4/1, Fcn5/1, Fcn6/1, Fcn7/1, Fcn1/1, Product/1
  Product/1 -> Add1/1
  Add1/1 -> Ceil/1
  ∠u/1 -> Add/1
  Multiport Switch1/1 -> theta'/1
  Fcn1/1 -> Multiport Switch1/8
  Constant8/1 -> Add1/2

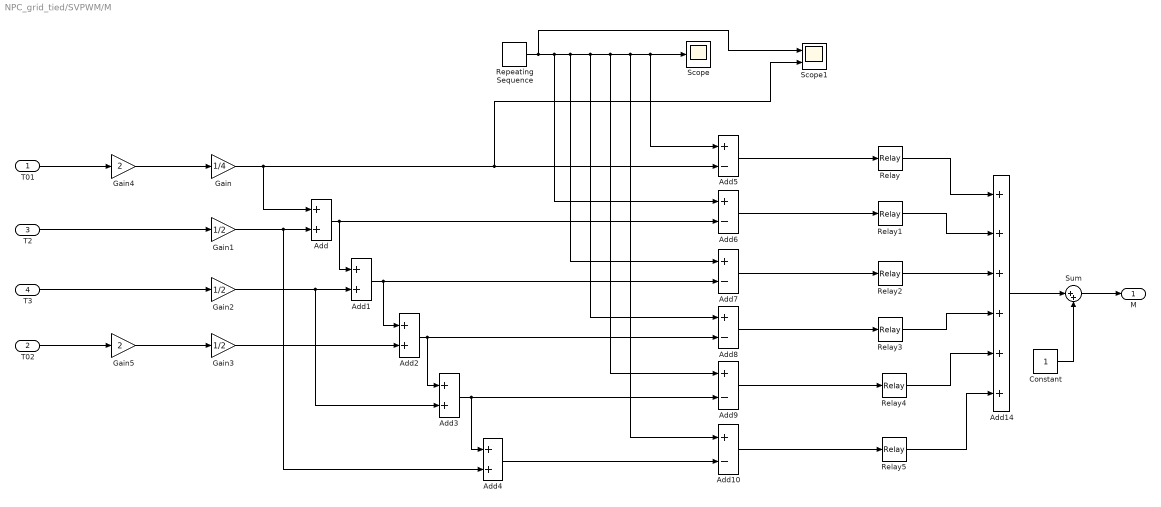
== system NPC_grid_tied/SVPWM/M ==
  T01 : Inport
  T02 : Inport  Port=2
  T2 : Inport  Port=3
  T3 : Inport  Port=4
  Add{,1..4} (5 alike) : Sum
  Add{5..10} (6 alike) : Sum  Inputs=+-
  Add14 : Sum  Inputs=++++++
  Constant : Constant
  Gain : Gain  Gain=1/4
  Gain1 : Gain  Gain=1/2
  Gain2 : Gain  Gain=1/2
  Gain3 : Gain  Gain=1/2
  Gain4 : Gain  Gain=2
  Gain5 : Gain  Gain=2
  Relay{,1..5} (6 alike) : Relay
  Repeating Sequence : simulink/Sources/Repeating Sequence  rep_seq_t=[0 1e-4]  rep_seq_y=[0 1e-4]
  Scope : Scope
  Scope1 : Scope  NumInputPorts=2
  Sum : Sum  Inputs=|++
  M : Outport  VectorParamsAs1DForOutWhenUnconnected=off
  wires:
  T01/1 -> Gain4/1
  Gain/1 -> Scope1/2, Add5/2, Add/1
  Add/1 -> Add6/2, Add1/1
  Add1/1 -> Add7/2, Add2/1
  Add2/1 -> Add8/2, Add3/1
  Add3/1 -> Add9/2, Add4/1
  Add4/1 -> Add10/2
  Gain3/1 -> Add2/2
  Gain1/1 -> Add/2, Add4/2
  Gain2/1 -> Add1/2, Add3/2
  Repeating Sequence/1 -> Scope1/1, Add6/1, Add7/1, Add8/1, Add9/1, Add10/1, Scope/1, Add5/1
  Add5/1 -> Relay/1
  Add6/1 -> Relay1/1
  Add7/1 -> Relay2/1
  Add8/1 -> Relay3/1
  Add9/1 -> Relay4/1
  Add10/1 -> Relay5/1
  Relay/1 -> Add14/1
  Relay2/1 -> Add14/3
  Relay1/1 -> Add14/2
  Relay3/1 -> Add14/4
  Relay4/1 -> Add14/5
  Relay5/1 -> Add14/6
  Constant/1 -> Sum/2
  Add14/1 -> Sum/1
  Sum/1 -> M/1
  Gain4/1 -> Gain/1
  T3/1 -> Gain2/1
  T2/1 -> Gain1/1
  T02/1 -> Gain5/1
  Gain5/1 -> Gain3/1

== system NPC_grid_tied/SVPWM/PI ==
  In1 : Inport
  Add : Sum
  Integrator : Integrator
  Ki : Gain  Gain=0.001
  Kp : Gain  Gain=1.6
  Saturation : Saturate
  Saturation1 : Saturate
  Out1 : Outport  VectorParamsAs1DForOutWhenUnconnected=off
  wires:
  Saturation1/1 -> Out1/1
  Add/1 -> Saturation1/1
  Saturation/1 -> Add/2
  Kp/1 -> Add/1
  In1/1 -> Ki/1, Kp/1
  Integrator/1 -> Saturation/1
  Ki/1 -> Integrator/1

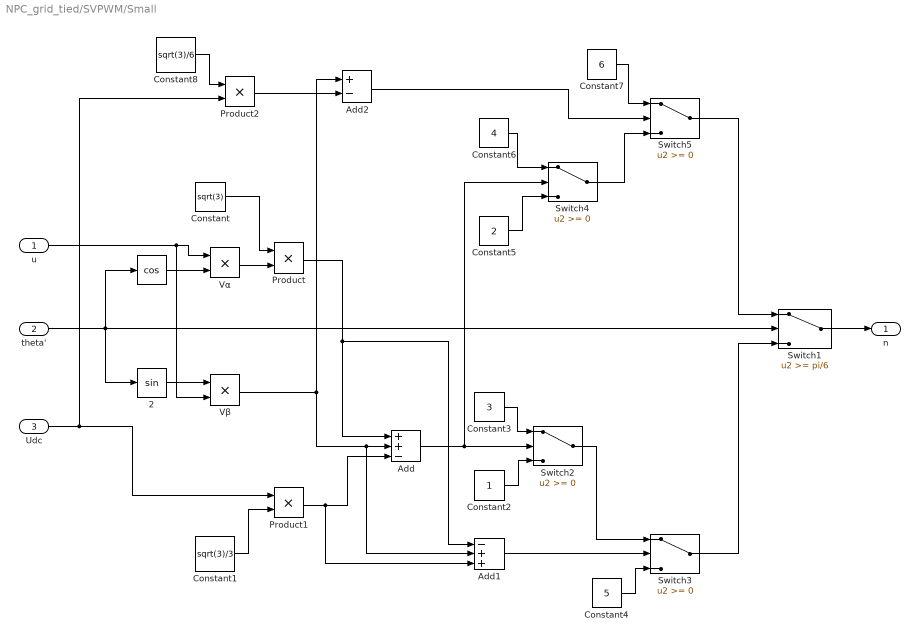
== system NPC_grid_tied/SVPWM/Small ==
  u : Inport
  theta' : Inport  Port=2
  Udc : Inport  Port=3
  " " : Trigonometry  Operator=cos
  " 2" : Trigonometry
  Add : Sum  Inputs=++-
  Add1 : Sum  Inputs=-++
  Add2 : Sum  Inputs=+-
  Constant : Constant  Value=sqrt(3)
  Constant1 : Constant  Value=sqrt(3)/3
  Constant2 : Constant
  Constant3 : Constant  Value=3
  Constant4 : Constant  Value=5
  Constant5 : Constant  Value=2
  Constant6 : Constant  Value=4
  Constant7 : Constant  Value=6
  Constant8 : Constant  Value=sqrt(3)/6
  Product : Product
  Product1 : Product
  Product2 : Product
  Switch1 : Switch  Threshold=pi/6
  Switch{2..5} (4 alike) : Switch
  Vα : Product
  Vβ : Product
  n : Outport  VectorParamsAs1DForOutWhenUnconnected=off
  wires:
  Constant/1 -> Product/1
  Switch2/1 -> Switch3/1
  Add1/1 -> Switch3/2
  Constant4/1 -> Switch3/3
  " 2"/1 -> Vβ/1
  Switch1/1 -> n/1
  Switch5/1 -> Switch1/1
  Constant5/1 -> Switch4/3
  Constant6/1 -> Switch4/1
  Add/1 -> Switch4/2, Switch2/2
  " "/1 -> Vα/2
  u/1 -> Vβ/2, Vα/1
  Vβ/1 -> Add2/1, Add1/2, Add/2
  Product/1 -> Add1/1, Add/1
  Product1/1 -> Add1/3, Add/3
  Vα/1 -> Product/2
  Constant3/1 -> Switch2/1
  Constant2/1 -> Switch2/3
  Constant7/1 -> Switch5/1
  Constant8/1 -> Product2/1
  Udc/1 -> Product2/2, Product1/1
  Add2/1 -> Switch5/2
  Product2/1 -> Add2/2
  Constant1/1 -> Product1/2
  Switch4/1 -> Switch5/3
  Switch3/1 -> Switch1/3
  theta'/1 -> Switch1/2, " 2"/1, " "/1

== system NPC_grid_tied/SVPWM/pulses ==
  state : Inport
  Add : Sum
  Constant : Constant
  Constant11 : Constant  Value=[1 1 0 0]
  Constant12 : Constant  Value=[0 0 1 1]
  Constant13 : Constant  Value=[0 1 1 0]
  Demux : Demux  Outputs=3
  Multiport Switch : MultiPortSwitch
  Multiport Switch1 : MultiPortSwitch
  Multiport Switch2 : MultiPortSwitch
  pulses1 : Outport  VectorParamsAs1DForOutWhenUnconnected=off
  pulses2 : Outport  Port=2  VectorParamsAs1DForOutWhenUnconnected=off
  pulses3 : Outport  Port=3  VectorParamsAs1DForOutWhenUnconnected=off
  wires:
  state/1 -> Add/1
  Constant/1 -> Add/2
  Add/1 -> Demux/1
  Demux/1 -> Multiport Switch/1
  Demux/2 -> Multiport Switch1/1
  Demux/3 -> Multiport Switch2/1
  Constant12/1 -> Multiport Switch/2, Multiport Switch1/2, Multiport Switch2/2
  Constant13/1 -> Multiport Switch/3, Multiport Switch1/3, Multiport Switch2/3
  Constant11/1 -> Multiport Switch/4, Multiport Switch1/4, Multiport Switch2/4
  Multiport Switch1/1 -> pulses2/1
  Multiport Switch/1 -> pulses1/1
  Multiport Switch2/1 -> pulses3/1

== system NPC_grid_tied/SVPWM/state ==
  n : Inport
  M : Inport  Port=2
  N : Inport  Port=3
  1 : Subsystem
  2 : Subsystem
  3 : Subsystem
  4 : Subsystem
  5 : Subsystem
  6 : Subsystem
  Multiport Switch : MultiPortSwitch  Inputs=6
  state : Outport  VectorParamsAs1DForOutWhenUnconnected=off
  wires:
  Multiport Switch/1 -> state/1
  N/1 -> Multiport Switch/1
  n/1 -> 1/1(n), 2/1(n), 3/1(n), 4/1(n), 5/1(n), 6/1(n)
  M/1 -> 1/2(M), 2/2(M), 3/2(M), 4/2(M), 5/2(M), 6/2(M)
  1/1(state) -> Multiport Switch/2
  2/1(state) -> Multiport Switch/3
  3/1(state) -> Multiport Switch/4
  4/1(state) -> Multiport Switch/5
  5/1(state) -> Multiport Switch/6
  6/1(state) -> Multiport Switch/7

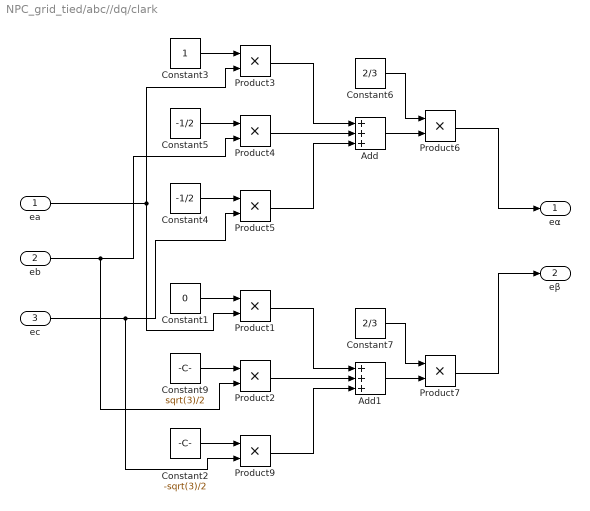
== system NPC_grid_tied/abc//dq/clark ==
  ea : Inport
  eb : Inport  Port=2
  ec : Inport  Port=3
  Add : Sum  Inputs=+++
  Add1 : Sum  Inputs=+++
  Constant1 : Constant  Value=0
  Constant2 : Constant  Value=-sqrt(3)/2
  Constant3 : Constant
  Constant4 : Constant  Value=-1/2
  Constant5 : Constant  Value=-1/2
  Constant6 : Constant  Value=2/3
  Constant7 : Constant  Value=2/3
  Constant9 : Constant  Value=sqrt(3)/2
  Product{1..7,9} (8 alike) : Product
  eα : Outport  VectorParamsAs1DForOutWhenUnconnected=off
  eβ : Outport  Port=2  VectorParamsAs1DForOutWhenUnconnected=off
  wires:
  Product5/1 -> Add/3
  eb/1 -> Product2/2, Product4/2
  Add1/1 -> Product7/2
  Constant7/1 -> Product7/1
  Product2/1 -> Add1/2
  Product4/1 -> Add/2
  Add/1 -> Product6/2
  Product6/1 -> eα/1
  Constant3/1 -> Product3/1
  Constant5/1 -> Product4/1
  ec/1 -> Product9/2, Product5/2
  ea/1 -> Product3/2, Product1/2
  Constant4/1 -> Product5/1
  Constant6/1 -> Product6/1
  Constant9/1 -> Product2/1
  Product3/1 -> Add/1
  Constant2/1 -> Product9/1
  Product9/1 -> Add1/3
  Product1/1 -> Add1/1
  Product7/1 -> eβ/1
  Constant1/1 -> Product1/1

== system NPC_grid_tied/abc//dq/park ==
  eα : Inport
  eβ : Inport  Port=2
  cos : Inport  Port=3
  sin : Inport  Port=4
  Add : Sum
  Add2 : Sum  Inputs=-+
  Product{,1..3} (4 alike) : Product
  ed : Outport  VectorParamsAs1DForOutWhenUnconnected=off
  eq : Outport  Port=2  VectorParamsAs1DForOutWhenUnconnected=off
  wires:
  Add2/1 -> eq/1
  Add/1 -> ed/1
  eα/1 -> Product2/1, Product/1
  cos/1 -> Product3/2, Product/2
  eβ/1 -> Product3/1, Product1/1
  sin/1 -> Product2/2, Product1/2
  Product/1 -> Add/1
  Product1/1 -> Add/2
  Product2/1 -> Add2/1
  Product3/1 -> Add2/2

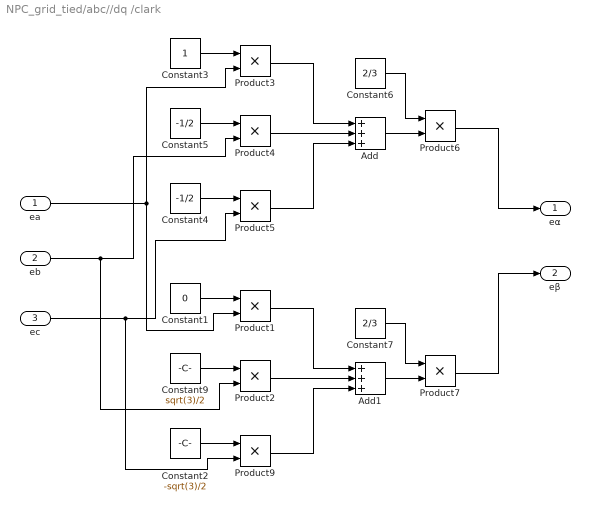
== system NPC_grid_tied/abc//dq /clark ==
  ea : Inport
  eb : Inport  Port=2
  ec : Inport  Port=3
  Add : Sum  Inputs=+++
  Add1 : Sum  Inputs=+++
  Constant1 : Constant  Value=0
  Constant2 : Constant  Value=-sqrt(3)/2
  Constant3 : Constant
  Constant4 : Constant  Value=-1/2
  Constant5 : Constant  Value=-1/2
  Constant6 : Constant  Value=2/3
  Constant7 : Constant  Value=2/3
  Constant9 : Constant  Value=sqrt(3)/2
  Product{1..7,9} (8 alike) : Product
  eα : Outport  VectorParamsAs1DForOutWhenUnconnected=off
  eβ : Outport  Port=2  VectorParamsAs1DForOutWhenUnconnected=off
  wires:
  Product5/1 -> Add/3
  eb/1 -> Product2/2, Product4/2
  Add1/1 -> Product7/2
  Constant7/1 -> Product7/1
  Product2/1 -> Add1/2
  Product4/1 -> Add/2
  Add/1 -> Product6/2
  Product6/1 -> eα/1
  Constant3/1 -> Product3/1
  Constant5/1 -> Product4/1
  ec/1 -> Product9/2, Product5/2
  ea/1 -> Product3/2, Product1/2
  Constant4/1 -> Product5/1
  Constant6/1 -> Product6/1
  Constant9/1 -> Product2/1
  Product3/1 -> Add/1
  Constant2/1 -> Product9/1
  Product9/1 -> Add1/3
  Product1/1 -> Add1/1
  Product7/1 -> eβ/1
  Constant1/1 -> Product1/1

== system NPC_grid_tied/abc//dq /park ==
  eα : Inport
  eβ : Inport  Port=2
  cos : Inport  Port=3
  sin : Inport  Port=4
  Add : Sum
  Add2 : Sum  Inputs=-+
  Product{,1..3} (4 alike) : Product
  ed : Outport  VectorParamsAs1DForOutWhenUnconnected=off
  eq : Outport  Port=2  VectorParamsAs1DForOutWhenUnconnected=off
  wires:
  Add2/1 -> eq/1
  Add/1 -> ed/1
  eα/1 -> Product2/1, Product/1
  cos/1 -> Product3/2, Product/2
  eβ/1 -> Product3/1, Product1/1
  sin/1 -> Product2/2, Product1/2
  Product/1 -> Add/1
  Product1/1 -> Add/2
  Product2/1 -> Add2/1
  Product3/1 -> Add2/2

== system NPC_grid_tied/SVPWM/state/1 ==
  n : Inport
  M : Inport  Port=2
  Multiport Switch : MultiPortSwitch  Inputs=6
  Subsystem10 : Subsystem
  Subsystem5 : Subsystem
  Subsystem6 : Subsystem
  Subsystem7 : Subsystem
  Subsystem8 : Subsystem
  Subsystem9 : Subsystem
  state : Outport  VectorParamsAs1DForOutWhenUnconnected=off
  wires:
  Multiport Switch/1 -> state/1
  n/1 -> Multiport Switch/1
  M/1 -> Subsystem5/1(M), Subsystem6/1(M), Subsystem7/1(M), Subsystem8/1(M), Subsystem9/1(M), Subsystem10/1(M)
  Subsystem5/1(state) -> Multiport Switch/2
  Subsystem6/1(state) -> Multiport Switch/3
  Subsystem7/1(state) -> Multiport Switch/4
  Subsystem8/1(state) -> Multiport Switch/5
  Subsystem9/1(state) -> Multiport Switch/6
  Subsystem10/1(state) -> Multiport Switch/7

== system NPC_grid_tied/SVPWM/state/2 ==
  n : Inport
  M : Inport  Port=2
  Multiport Switch : MultiPortSwitch  Inputs=6
  Subsystem10 : Subsystem
  Subsystem5 : Subsystem
  Subsystem6 : Subsystem
  Subsystem7 : Subsystem
  Subsystem8 : Subsystem
  Subsystem9 : Subsystem
  state : Outport  VectorParamsAs1DForOutWhenUnconnected=off
  wires:
  Subsystem10/1(state) -> Multiport Switch/7
  Subsystem9/1(state) -> Multiport Switch/6
  Subsystem8/1(state) -> Multiport Switch/5
  Subsystem7/1(state) -> Multiport Switch/4
  Subsystem6/1(state) -> Multiport Switch/3
  Subsystem5/1(state) -> Multiport Switch/2
  M/1 -> Subsystem10/1(M), Subsystem9/1(M), Subsystem8/1(M), Subsystem7/1(M), Subsystem6/1(M), Subsystem5/1(M)
  n/1 -> Multiport Switch/1
  Multiport Switch/1 -> state/1

== system NPC_grid_tied/SVPWM/state/3 ==
  n : Inport
  M : Inport  Port=2
  Multiport Switch : MultiPortSwitch  Inputs=6
  Subsystem10 : Subsystem
  Subsystem5 : Subsystem
  Subsystem6 : Subsystem
  Subsystem7 : Subsystem
  Subsystem8 : Subsystem
  Subsystem9 : Subsystem
  state : Outport  VectorParamsAs1DForOutWhenUnconnected=off
  wires:
  Multiport Switch/1 -> state/1
  n/1 -> Multiport Switch/1
  M/1 -> Subsystem5/1(M), Subsystem6/1(M), Subsystem7/1(M), Subsystem8/1(M), Subsystem9/1(M), Subsystem10/1(M)
  Subsystem5/1(state) -> Multiport Switch/2
  Subsystem6/1(state) -> Multiport Switch/3
  Subsystem7/1(state) -> Multiport Switch/4
  Subsystem8/1(state) -> Multiport Switch/5
  Subsystem9/1(state) -> Multiport Switch/6
  Subsystem10/1(state) -> Multiport Switch/7

== system NPC_grid_tied/SVPWM/state/4 ==
  n : Inport
  M : Inport  Port=2
  Multiport Switch : MultiPortSwitch  Inputs=6
  Subsystem10 : Subsystem
  Subsystem5 : Subsystem
  Subsystem6 : Subsystem
  Subsystem7 : Subsystem
  Subsystem8 : Subsystem
  Subsystem9 : Subsystem
  state : Outport  VectorParamsAs1DForOutWhenUnconnected=off
  wires:
  Subsystem10/1(state) -> Multiport Switch/7
  Subsystem9/1(state) -> Multiport Switch/6
  Subsystem8/1(state) -> Multiport Switch/5
  Subsystem7/1(state) -> Multiport Switch/4
  Subsystem6/1(state) -> Multiport Switch/3
  Subsystem5/1(state) -> Multiport Switch/2
  M/1 -> Subsystem10/1(M), Subsystem9/1(M), Subsystem8/1(M), Subsystem7/1(M), Subsystem6/1(M), Subsystem5/1(M)
  n/1 -> Multiport Switch/1
  Multiport Switch/1 -> state/1

== system NPC_grid_tied/SVPWM/state/5 ==
  n : Inport
  M : Inport  Port=2
  Multiport Switch : MultiPortSwitch  Inputs=6
  Subsystem10 : Subsystem
  Subsystem5 : Subsystem
  Subsystem6 : Subsystem
  Subsystem7 : Subsystem
  Subsystem8 : Subsystem
  Subsystem9 : Subsystem
  state : Outport  VectorParamsAs1DForOutWhenUnconnected=off
  wires:
  Multiport Switch/1 -> state/1
  n/1 -> Multiport Switch/1
  M/1 -> Subsystem5/1(M), Subsystem7/1(M), Subsystem8/1(M), Subsystem9/1(M), Subsystem10/1(M), Subsystem6/1(M)
  Subsystem5/1(state) -> Multiport Switch/2
  Subsystem6/1(state) -> Multiport Switch/3
  Subsystem7/1(state) -> Multiport Switch/4
  Subsystem8/1(state) -> Multiport Switch/5
  Subsystem9/1(state) -> Multiport Switch/6
  Subsystem10/1(state) -> Multiport Switch/7

== system NPC_grid_tied/SVPWM/state/6 ==
  n : Inport
  M : Inport  Port=2
  Multiport Switch : MultiPortSwitch  Inputs=6
  Subsystem10 : Subsystem
  Subsystem5 : Subsystem
  Subsystem6 : Subsystem
  Subsystem7 : Subsystem
  Subsystem8 : Subsystem
  Subsystem9 : Subsystem
  state : Outport  VectorParamsAs1DForOutWhenUnconnected=off
  wires:
  Subsystem10/1(state) -> Multiport Switch/7
  Subsystem9/1(state) -> Multiport Switch/6
  Subsystem8/1(state) -> Multiport Switch/5
  Subsystem7/1(state) -> Multiport Switch/4
  Subsystem6/1(state) -> Multiport Switch/3
  Subsystem5/1(state) -> Multiport Switch/2
  M/1 -> Subsystem10/1(M), Subsystem9/1(M), Subsystem8/1(M), Subsystem7/1(M), Subsystem6/1(M), Subsystem5/1(M)
  n/1 -> Multiport Switch/1
  Multiport Switch/1 -> state/1

== system NPC_grid_tied/SVPWM/state/1/Subsystem10 ==
  M : Inport
  Constant : Constant  Value=[1 1 0]
  Constant1 : Constant  Value=[2 1 0]
  Constant2 : Constant  Value=[2 2 0]
  Constant3 : Constant  Value=[2 2 1]
  Constant4 : Constant  Value=[2 1 0]
  Constant5 : Constant  Value=[2 2 0]
  Constant6 : Constant  Value=[1 1 0]
  Multiport Switch : MultiPortSwitch  Inputs=7
  state : Outport  VectorParamsAs1DForOutWhenUnconnected=off
  wires:
  Constant6/1 -> Multiport Switch/8
  Constant4/1 -> Multiport Switch/7
  Constant5/1 -> Multiport Switch/6
  Constant3/1 -> Multiport Switch/5
  Constant2/1 -> Multiport Switch/4
  Constant1/1 -> Multiport Switch/3
  Constant/1 -> Multiport Switch/2
  M/1 -> Multiport Switch/1
  Multiport Switch/1 -> state/1

== system NPC_grid_tied/SVPWM/state/1/Subsystem5 ==
  M : Inport
  Constant : Constant  Value=[1 0 0]
  Constant1 : Constant  Value=[1 1 0]
  Constant2 : Constant  Value=[1 1 1]
  Constant3 : Constant  Value=[2 1 1]
  Constant4 : Constant  Value=[1 1 0]
  Constant5 : Constant  Value=[1 1 1]
  Constant6 : Constant  Value=[1 0 0]
  Multiport Switch : MultiPortSwitch  Inputs=7
  state : Outport  VectorParamsAs1DForOutWhenUnconnected=off
  wires:
  Multiport Switch/1 -> state/1
  M/1 -> Multiport Switch/1
  Constant/1 -> Multiport Switch/2
  Constant1/1 -> Multiport Switch/3
  Constant2/1 -> Multiport Switch/4
  Constant3/1 -> Multiport Switch/5
  Constant5/1 -> Multiport Switch/6
  Constant4/1 -> Multiport Switch/7
  Constant6/1 -> Multiport Switch/8

== system NPC_grid_tied/SVPWM/state/1/Subsystem6 ==
  M : Inport
  Constant : Constant  Value=[1 1 0]
  Constant1 : Constant  Value=[1 1 1]
  Constant2 : Constant  Value=[2 1 1]
  Constant3 : Constant  Value=[2 2 1]
  Constant4 : Constant  Value=[1 1 1]
  Constant5 : Constant  Value=[2 1 1]
  Constant6 : Constant  Value=[1 1 0]
  Multiport Switch : MultiPortSwitch  Inputs=7
  state : Outport  VectorParamsAs1DForOutWhenUnconnected=off
  wires:
  Constant6/1 -> Multiport Switch/8
  Constant4/1 -> Multiport Switch/7
  Constant5/1 -> Multiport Switch/6
  Constant3/1 -> Multiport Switch/5
  Constant2/1 -> Multiport Switch/4
  Constant1/1 -> Multiport Switch/3
  Constant/1 -> Multiport Switch/2
  M/1 -> Multiport Switch/1
  Multiport Switch/1 -> state/1

== system NPC_grid_tied/SVPWM/state/1/Subsystem7 ==
  M : Inport
  Constant : Constant  Value=[1 0 0]
  Constant1 : Constant  Value=[1 1 0]
  Constant2 : Constant  Value=[2 1 0]
  Constant3 : Constant  Value=[2 1 1]
  Constant4 : Constant  Value=[1 1 0]
  Constant5 : Constant  Value=[2 1 0]
  Constant6 : Constant  Value=[1 0 0]
  Multiport Switch : MultiPortSwitch  Inputs=7
  state : Outport  VectorParamsAs1DForOutWhenUnconnected=off
  wires:
  Multiport Switch/1 -> state/1
  M/1 -> Multiport Switch/1
  Constant/1 -> Multiport Switch/2
  Constant1/1 -> Multiport Switch/3
  Constant2/1 -> Multiport Switch/4
  Constant3/1 -> Multiport Switch/5
  Constant5/1 -> Multiport Switch/6
  Constant4/1 -> Multiport Switch/7
  Constant6/1 -> Multiport Switch/8

== system NPC_grid_tied/SVPWM/state/1/Subsystem8 ==
  M : Inport
  Constant : Constant  Value=[1 1 0]
  Constant1 : Constant  Value=[2 1 0]
  Constant2 : Constant  Value=[2 1 1]
  Constant3 : Constant  Value=[2 2 1]
  Constant4 : Constant  Value=[2 1 0]
  Constant5 : Constant  Value=[2 1 1]
  Constant6 : Constant  Value=[1 1 0]
  Multiport Switch : MultiPortSwitch  Inputs=7
  state : Outport  VectorParamsAs1DForOutWhenUnconnected=off
  wires:
  Constant6/1 -> Multiport Switch/8
  Constant4/1 -> Multiport Switch/7
  Constant5/1 -> Multiport Switch/6
  Constant3/1 -> Multiport Switch/5
  Constant2/1 -> Multiport Switch/4
  Constant1/1 -> Multiport Switch/3
  Constant/1 -> Multiport Switch/2
  M/1 -> Multiport Switch/1
  Multiport Switch/1 -> state/1

== system NPC_grid_tied/SVPWM/state/1/Subsystem9 ==
  M : Inport
  Constant : Constant  Value=[1 0 0]
  Constant1 : Constant  Value=[2 0 0]
  Constant2 : Constant  Value=[2 1 0]
  Constant3 : Constant  Value=[2 1 1]
  Constant4 : Constant  Value=[2 0 0]
  Constant5 : Constant  Value=[2 1 0]
  Constant6 : Constant  Value=[1 0 0]
  Multiport Switch : MultiPortSwitch  Inputs=7
  state : Outport  VectorParamsAs1DForOutWhenUnconnected=off
  wires:
  Multiport Switch/1 -> state/1
  M/1 -> Multiport Switch/1
  Constant/1 -> Multiport Switch/2
  Constant1/1 -> Multiport Switch/3
  Constant2/1 -> Multiport Switch/4
  Constant3/1 -> Multiport Switch/5
  Constant5/1 -> Multiport Switch/6
  Constant4/1 -> Multiport Switch/7
  Constant6/1 -> Multiport Switch/8

== system NPC_grid_tied/SVPWM/state/2/Subsystem10 ==
  M : Inport
  Constant : Constant  Value=[0 1 0]
  Constant1 : Constant  Value=[0 2 0]
  Constant2 : Constant  Value=[1 2 0]
  Constant3 : Constant  Value=[1 2 1]
  Constant4 : Constant  Value=[0 2 0]
  Constant5 : Constant  Value=[1 2 0]
  Constant6 : Constant  Value=[0 1 0]
  Multiport Switch : MultiPortSwitch  Inputs=7
  state : Outport  VectorParamsAs1DForOutWhenUnconnected=off
  wires:
  Multiport Switch/1 -> state/1
  M/1 -> Multiport Switch/1
  Constant/1 -> Multiport Switch/2
  Constant1/1 -> Multiport Switch/3
  Constant2/1 -> Multiport Switch/4
  Constant3/1 -> Multiport Switch/5
  Constant5/1 -> Multiport Switch/6
  Constant4/1 -> Multiport Switch/7
  Constant6/1 -> Multiport Switch/8

== system NPC_grid_tied/SVPWM/state/2/Subsystem5 ==
  M : Inport
  Constant : Constant  Value=[1 1 0]
  Constant1 : Constant  Value=[1 1 1]
  Constant2 : Constant  Value=[1 2 1]
  Constant3 : Constant  Value=[2 2 1]
  Constant4 : Constant  Value=[1 1 1]
  Constant5 : Constant  Value=[1 2 1]
  Constant6 : Constant  Value=[1 1 0]
  Multiport Switch : MultiPortSwitch  Inputs=7
  state : Outport  VectorParamsAs1DForOutWhenUnconnected=off
  wires:
  Constant6/1 -> Multiport Switch/8
  Constant4/1 -> Multiport Switch/7
  Constant5/1 -> Multiport Switch/6
  Constant3/1 -> Multiport Switch/5
  Constant2/1 -> Multiport Switch/4
  Constant1/1 -> Multiport Switch/3
  Constant/1 -> Multiport Switch/2
  M/1 -> Multiport Switch/1
  Multiport Switch/1 -> state/1
